simulink model "sampleModel7126_pp_1_1"  (R2018a)
settings: Solver=VariableStepAuto  StartTime=0.0  StopTime=10.0  RelTol=1e-3
undefined symbols (not defined in the file): DiscIntNeverNeededParam
libraries: simulink x367
(part 12 of 12)

== system sampleModel7126_pp_1_1/cfblk284/cfblk10/emi_600 ==
  Action Port : ActionPort  ActionType=else
  emi_601 : Assertion

== system sampleModel7126_pp_1_1/cfblk284/cfblk11/cfblk10 ==
  emi_481 : Inport
  emi_482 : Inport  Port=2
  Action Port : ActionPort  ActionType=then
  cfblk10 : simulink/Continuous/PID Controller (2DOF)  Controller=PID  TimeDomain=Discrete-time  SampleTime=-1  IntegratorMethod=Forward Euler  FilterMethod=Forward Euler  Form=Parallel  UseFilter=on  ControllerParametersSource=internal  P=1  I=1  D=0  N=100  b=1  c=1  InitialConditionSource=internal  InitialConditionForIntegrator=0  InitialConditionForFilter=0  ExternalReset=none  LimitOutput=off  UpperSaturationLimit=inf  LowerSaturationLimit=-inf  LinearizeAsGain=off  AntiWindupMode=none  Kb=1  TrackingMode=off  Kt=1  PParamMin=[]  PParamMax=[]  IParamMin=[]  IParamMax=[]  DParamMin=[]  DParamMax=[]  NParamMin=[]  NParamMax=[]  bParamMin=[]  bParamMax=[]  cParamMin=[]  cParamMax=[]  KbParamMin=[]  KbParamMax=[]  KtParamMin=[]  KtParamMax=[]  POutMin=[]  POutMax=[]  IOutMin=[]  IOutMax=[]  DOutMin=[]  DOutMax=[]  NOutMin=[]  NOutMax=[]  bOutMin=[]  bOutMax=[]  cOutMin=[]  cOutMax=[]  KbOutMin=[]  KbOutMax=[]  KtOutMin=[]  KtOutMax=[]  IntegratorOutMin=[]  IntegratorOutMax=[]  FilterOutMin=[]  FilterOutMax=[]  SumOutMin=[]  SumOutMax=[]  Sum1OutMin=[]  Sum1OutMax=[]  Sum2OutMin=[]  Sum2OutMax=[]  Sum3OutMin=[]  Sum3OutMax=[]  SumI1OutMin=[]  SumI1OutMax=[]  SumI2OutMin=[]  SumI2OutMax=[]  SumI3OutMin=[]  SumI3OutMax=[]  SumDOutMin=[]  SumDOutMax=[]  SaturationOutMin=[]  SaturationOutMax=[]  IntegratorContinuousStateAttributes=''  IntegratorStateMustResolveToSignalObject=off  IntegratorRTWStateStorageClass=Auto  FilterContinuousStateAttributes=''  FilterStateMustResolveToSignalObject=off  FilterRTWStateStorageClass=Auto  DifferentiatorICPrevScaledInput=0  DifferentiatorOutMin=[]  DifferentiatorOutMax=[]  FilterDiffOutCoefMin=[]  FilterDiffOutCoefMax=[]  SumDenOutMin=[]  SumDenOutMax=[]  SumNumOutMin=[]  SumNumOutMax=[]  ReciprocalOutMin=[]  ReciprocalOutMax=[]  DivideOutMin=[]  DivideOutMax=[]  TunerSelectOption=Transfer Function Based (PID Tuner App)
  emi_483 : Outport
  wires:
  emi_481/1 -> cfblk10/1
  emi_482/1 -> cfblk10/2
  cfblk10/1 -> emi_483/1

== system sampleModel7126_pp_1_1/cfblk284/cfblk11/cfblk11 ==
  emi_1583 : Inport
  Action Port : ActionPort  ActionType=then
  cfblk11 : simulink/Discrete/Transfer Fcn Real Zero  ZeroZ=0.75  ICPrevInput=0.0  DoSatur=off
      settings: SourceProductName=Simulink  SourceProductBaseCode=SL
  emi_1584 : Outport
  wires:
  emi_1583/1 -> cfblk11/1
  cfblk11/1 -> emi_1584/1

== system sampleModel7126_pp_1_1/cfblk284/cfblk11/cfblk4 ==
  emi_1611 : Inport
  Action Port : ActionPort  ActionType=then
  cfblk4 : simulink/Discrete/Transfer Fcn Real Zero  ZeroZ=0.75  ICPrevInput=0.0  DoSatur=off
      settings: SourceProductName=Simulink  SourceProductBaseCode=SL
  emi_1612 : Outport
  wires:
  emi_1611/1 -> cfblk4/1
  cfblk4/1 -> emi_1612/1

== system sampleModel7126_pp_1_1/cfblk284/cfblk11/cfblk8 ==
  emi_1461 : Inport
  emi_1462 : Inport  Port=2
  Action Port : ActionPort  ActionType=then
  cfblk8 : simulink/Continuous/PID Controller (2DOF)  Controller=PID  TimeDomain=Discrete-time  SampleTime=-1  IntegratorMethod=Forward Euler  FilterMethod=Forward Euler  Form=Parallel  UseFilter=on  ControllerParametersSource=internal  P=1  I=1  D=0  N=100  b=1  c=1  InitialConditionSource=internal  InitialConditionForIntegrator=0  InitialConditionForFilter=0  ExternalReset=none  LimitOutput=off  UpperSaturationLimit=inf  LowerSaturationLimit=-inf  LinearizeAsGain=off  AntiWindupMode=none  Kb=1  TrackingMode=off  Kt=1  PParamMin=[]  PParamMax=[]  IParamMin=[]  IParamMax=[]  DParamMin=[]  DParamMax=[]  NParamMin=[]  NParamMax=[]  bParamMin=[]  bParamMax=[]  cParamMin=[]  cParamMax=[]  KbParamMin=[]  KbParamMax=[]  KtParamMin=[]  KtParamMax=[]  POutMin=[]  POutMax=[]  IOutMin=[]  IOutMax=[]  DOutMin=[]  DOutMax=[]  NOutMin=[]  NOutMax=[]  bOutMin=[]  bOutMax=[]  cOutMin=[]  cOutMax=[]  KbOutMin=[]  KbOutMax=[]  KtOutMin=[]  KtOutMax=[]  IntegratorOutMin=[]  IntegratorOutMax=[]  FilterOutMin=[]  FilterOutMax=[]  SumOutMin=[]  SumOutMax=[]  Sum1OutMin=[]  Sum1OutMax=[]  Sum2OutMin=[]  Sum2OutMax=[]  Sum3OutMin=[]  Sum3OutMax=[]  SumI1OutMin=[]  SumI1OutMax=[]  SumI2OutMin=[]  SumI2OutMax=[]  SumI3OutMin=[]  SumI3OutMax=[]  SumDOutMin=[]  SumDOutMax=[]  SaturationOutMin=[]  SaturationOutMax=[]  IntegratorContinuousStateAttributes=''  IntegratorStateMustResolveToSignalObject=off  IntegratorRTWStateStorageClass=Auto  FilterContinuousStateAttributes=''  FilterStateMustResolveToSignalObject=off  FilterRTWStateStorageClass=Auto  DifferentiatorICPrevScaledInput=0  DifferentiatorOutMin=[]  DifferentiatorOutMax=[]  FilterDiffOutCoefMin=[]  FilterDiffOutCoefMax=[]  SumDenOutMin=[]  SumDenOutMax=[]  SumNumOutMin=[]  SumNumOutMax=[]  ReciprocalOutMin=[]  ReciprocalOutMax=[]  DivideOutMin=[]  DivideOutMax=[]  TunerSelectOption=Transfer Function Based (PID Tuner App)
  emi_1463 : Outport
  wires:
  emi_1461/1 -> cfblk8/1
  emi_1462/1 -> cfblk8/2
  cfblk8/1 -> emi_1463/1

== system sampleModel7126_pp_1_1/cfblk284/cfblk11/emi_1464 ==
  Action Port : ActionPort  ActionType=else
  emi_1465 : Assertion

== system sampleModel7126_pp_1_1/cfblk284/cfblk11/emi_1585 ==
  Action Port : ActionPort  ActionType=else
  emi_1586 : Assertion

== system sampleModel7126_pp_1_1/cfblk284/cfblk11/emi_1613 ==
  Action Port : ActionPort  ActionType=else
  emi_1614 : Assertion

== system sampleModel7126_pp_1_1/cfblk284/cfblk11/emi_484 ==
  Action Port : ActionPort  ActionType=else
  emi_485 : Assertion

== system sampleModel7126_pp_1_1/cfblk289/cfblk10/cfblk4 ==
  emi_981 : Inport
  Action Port : ActionPort  ActionType=then
  cfblk4 : DiscreteIntegrator  SampleTime=-1  OutDataTypeStr=double  ICPrevOutput=DiscIntNeverNeededParam  ICPrevScaledInput=DiscIntNeverNeededParam
  emi_982 : Outport
  wires:
  emi_981/1 -> cfblk4/1
  cfblk4/1 -> emi_982/1

== system sampleModel7126_pp_1_1/cfblk289/cfblk10/cfblk5 ==
  emi_974 : Inport
  Action Port : ActionPort  ActionType=then
  cfblk5 : simulink/Discrete/Transfer Fcn Real Zero  ZeroZ=0.75  ICPrevInput=0.0  DoSatur=off
      settings: SourceProductName=Simulink  SourceProductBaseCode=SL
  emi_975 : Outport
  wires:
  emi_974/1 -> cfblk5/1
  cfblk5/1 -> emi_975/1

== system sampleModel7126_pp_1_1/cfblk289/cfblk10/cfblk7 ==
  emi_1405 : Inport
  Action Port : ActionPort  ActionType=then
  cfblk7 : Delay
  emi_1406 : Outport
  wires:
  emi_1405/1 -> cfblk7/1
  cfblk7/1 -> emi_1406/1

== system sampleModel7126_pp_1_1/cfblk289/cfblk10/cfblk9 ==
  emi_584 : Inport
  Action Port : ActionPort  ActionType=then
  cfblk9 : DiscreteFilter
  emi_585 : Outport
  wires:
  emi_584/1 -> cfblk9/1
  cfblk9/1 -> emi_585/1

== system sampleModel7126_pp_1_1/cfblk289/cfblk10/emi_1407 ==
  Action Port : ActionPort  ActionType=else
  emi_1408 : Assertion

== system sampleModel7126_pp_1_1/cfblk289/cfblk10/emi_586 ==
  Action Port : ActionPort  ActionType=else
  emi_587 : Assertion

== system sampleModel7126_pp_1_1/cfblk289/cfblk10/emi_976 ==
  Action Port : ActionPort  ActionType=else
  emi_977 : Assertion

== system sampleModel7126_pp_1_1/cfblk289/cfblk10/emi_983 ==
  Action Port : ActionPort  ActionType=else
  emi_984 : Assertion

== system sampleModel7126_pp_1_1/cfblk289/cfblk9/cfblk10 ==
  emi_818 : Inport
  Action Port : ActionPort  ActionType=then
  cfblk10 : DiscreteFir
  emi_819 : Outport
  wires:
  emi_818/1 -> cfblk10/1
  cfblk10/1 -> emi_819/1

== system sampleModel7126_pp_1_1/cfblk289/cfblk9/cfblk12 ==
  emi_1667 : Inport
  Action Port : ActionPort  ActionType=then
  cfblk12 : DiscreteTransferFcn
  emi_1668 : Outport
  wires:
  emi_1667/1 -> cfblk12/1
  cfblk12/1 -> emi_1668/1

== system sampleModel7126_pp_1_1/cfblk289/cfblk9/cfblk15 ==
  emi_1246 : Inport
  emi_1247 : Inport  Port=2
  Action Port : ActionPort  ActionType=then
  cfblk15 : simulink/Continuous/PID Controller (2DOF)  Controller=PID  TimeDomain=Discrete-time  SampleTime=-1  IntegratorMethod=Forward Euler  FilterMethod=Forward Euler  Form=Parallel  UseFilter=on  ControllerParametersSource=internal  P=1  I=1  D=0  N=100  b=1  c=1  InitialConditionSource=internal  InitialConditionForIntegrator=0  InitialConditionForFilter=0  ExternalReset=none  LimitOutput=off  UpperSaturationLimit=inf  LowerSaturationLimit=-inf  LinearizeAsGain=off  AntiWindupMode=none  Kb=1  TrackingMode=off  Kt=1  PParamMin=[]  PParamMax=[]  IParamMin=[]  IParamMax=[]  DParamMin=[]  DParamMax=[]  NParamMin=[]  NParamMax=[]  bParamMin=[]  bParamMax=[]  cParamMin=[]  cParamMax=[]  KbParamMin=[]  KbParamMax=[]  KtParamMin=[]  KtParamMax=[]  POutMin=[]  POutMax=[]  IOutMin=[]  IOutMax=[]  DOutMin=[]  DOutMax=[]  NOutMin=[]  NOutMax=[]  bOutMin=[]  bOutMax=[]  cOutMin=[]  cOutMax=[]  KbOutMin=[]  KbOutMax=[]  KtOutMin=[]  KtOutMax=[]  IntegratorOutMin=[]  IntegratorOutMax=[]  FilterOutMin=[]  FilterOutMax=[]  SumOutMin=[]  SumOutMax=[]  Sum1OutMin=[]  Sum1OutMax=[]  Sum2OutMin=[]  Sum2OutMax=[]  Sum3OutMin=[]  Sum3OutMax=[]  SumI1OutMin=[]  SumI1OutMax=[]  SumI2OutMin=[]  SumI2OutMax=[]  SumI3OutMin=[]  SumI3OutMax=[]  SumDOutMin=[]  SumDOutMax=[]  SaturationOutMin=[]  SaturationOutMax=[]  IntegratorContinuousStateAttributes=''  IntegratorStateMustResolveToSignalObject=off  IntegratorRTWStateStorageClass=Auto  FilterContinuousStateAttributes=''  FilterStateMustResolveToSignalObject=off  FilterRTWStateStorageClass=Auto  DifferentiatorICPrevScaledInput=0  DifferentiatorOutMin=[]  DifferentiatorOutMax=[]  FilterDiffOutCoefMin=[]  FilterDiffOutCoefMax=[]  SumDenOutMin=[]  SumDenOutMax=[]  SumNumOutMin=[]  SumNumOutMax=[]  ReciprocalOutMin=[]  ReciprocalOutMax=[]  DivideOutMin=[]  DivideOutMax=[]  TunerSelectOption=Transfer Function Based (PID Tuner App)
  emi_1248 : Outport
  wires:
  emi_1246/1 -> cfblk15/1
  emi_1247/1 -> cfblk15/2
  cfblk15/1 -> emi_1248/1

== system sampleModel7126_pp_1_1/cfblk289/cfblk9/cfblk8 ==
  emi_1433 : Inport
  Action Port : ActionPort  ActionType=then
  cfblk8 : Delay
  emi_1434 : Outport
  wires:
  emi_1433/1 -> cfblk8/1
  cfblk8/1 -> emi_1434/1

== system sampleModel7126_pp_1_1/cfblk289/cfblk9/cfblk9 ==
  emi_1254 : Inport
  Action Port : ActionPort  ActionType=then
  cfblk9 : DiscreteFir
  emi_1255 : Outport
  wires:
  emi_1254/1 -> cfblk9/1
  cfblk9/1 -> emi_1255/1

== system sampleModel7126_pp_1_1/cfblk289/cfblk9/emi_1249 ==
  Action Port : ActionPort  ActionType=else
  emi_1250 : Assertion

== system sampleModel7126_pp_1_1/cfblk289/cfblk9/emi_1256 ==
  Action Port : ActionPort  ActionType=else
  emi_1257 : Assertion

== system sampleModel7126_pp_1_1/cfblk289/cfblk9/emi_1435 ==
  Action Port : ActionPort  ActionType=else
  emi_1436 : Assertion

== system sampleModel7126_pp_1_1/cfblk289/cfblk9/emi_1669 ==
  Action Port : ActionPort  ActionType=else
  emi_1670 : Assertion

== system sampleModel7126_pp_1_1/cfblk289/cfblk9/emi_820 ==
  Action Port : ActionPort  ActionType=else
  emi_821 : Assertion

== system sampleModel7126_pp_1_1/cfblk292/cfblk14/cfblk3 ==
  emi_1426 : Inport
  Action Port : ActionPort  ActionType=then
  cfblk3 : DiscreteFir
  emi_1427 : Outport
  wires:
  emi_1426/1 -> cfblk3/1
  cfblk3/1 -> emi_1427/1

== system sampleModel7126_pp_1_1/cfblk292/cfblk14/cfblk4 ==
  emi_351 : Inport
  Action Port : ActionPort  ActionType=then
  cfblk4 : simulink/Discrete/Transfer Fcn Real Zero  ZeroZ=0.75  ICPrevInput=0.0  DoSatur=off
      settings: SourceProductName=Simulink  SourceProductBaseCode=SL
  emi_352 : Outport
  wires:
  emi_351/1 -> cfblk4/1
  cfblk4/1 -> emi_352/1

== system sampleModel7126_pp_1_1/cfblk292/cfblk14/emi_1428 ==
  Action Port : ActionPort  ActionType=else
  emi_1429 : Assertion

== system sampleModel7126_pp_1_1/cfblk292/cfblk14/emi_353 ==
  Action Port : ActionPort  ActionType=else
  emi_354 : Assertion

== system sampleModel7126_pp_1_1/cfblk292/cfblk15/cfblk13 ==
  emi_1412 : Inport
  Action Port : ActionPort  ActionType=then
  cfblk13 : Delay
  emi_1413 : Outport
  wires:
  emi_1412/1 -> cfblk13/1
  cfblk13/1 -> emi_1413/1

== system sampleModel7126_pp_1_1/cfblk292/cfblk15/cfblk3 ==
  emi_453 : Inport
  Action Port : ActionPort  ActionType=then
  cfblk3 : simulink/Continuous/PID Controller  Controller=PID  TimeDomain=Discrete-time  SampleTime=-1  IntegratorMethod=Forward Euler  FilterMethod=Forward Euler  Form=Parallel  UseFilter=on  ControllerParametersSource=internal  P=1  I=1  D=0  N=100  InitialConditionSource=internal  InitialConditionForIntegrator=0  InitialConditionForFilter=0  ExternalReset=none  LimitOutput=off  UpperSaturationLimit=inf  LowerSaturationLimit=-inf  LinearizeAsGain=off  AntiWindupMode=none  Kb=1  TrackingMode=off  Kt=1  PParamMin=[]  PParamMax=[]  IParamMin=[]  IParamMax=[]  DParamMin=[]  DParamMax=[]  NParamMin=[]  NParamMax=[]  KbParamMin=[]  KbParamMax=[]  KtParamMin=[]  KtParamMax=[]  POutMin=[]  POutMax=[]  IOutMin=[]  IOutMax=[]  DOutMin=[]  DOutMax=[]  NOutMin=[]  NOutMax=[]  KbOutMin=[]  KbOutMax=[]  KtOutMin=[]  KtOutMax=[]  IntegratorOutMin=[]  IntegratorOutMax=[]  FilterOutMin=[]  FilterOutMax=[]  SumOutMin=[]  SumOutMax=[]  SumI1OutMin=[]  SumI1OutMax=[]  SumI2OutMin=[]  SumI2OutMax=[]  SumI3OutMin=[]  SumI3OutMax=[]  SumDOutMin=[]  SumDOutMax=[]  SaturationOutMin=[]  SaturationOutMax=[]  IntegratorContinuousStateAttributes=''  IntegratorStateMustResolveToSignalObject=off  IntegratorRTWStateStorageClass=Auto  FilterContinuousStateAttributes=''  FilterStateMustResolveToSignalObject=off  FilterRTWStateStorageClass=Auto  DifferentiatorICPrevScaledInput=0  DifferentiatorOutMin=[]  DifferentiatorOutMax=[]  FilterDiffOutCoefMin=[]  FilterDiffOutCoefMax=[]  SumDenOutMin=[]  SumDenOutMax=[]  SumNumOutMin=[]  SumNumOutMax=[]  ReciprocalOutMin=[]  ReciprocalOutMax=[]  DivideOutMin=[]  DivideOutMax=[]  TunerSelectOption=Transfer Function Based (PID Tuner App)
  emi_454 : Outport
  wires:
  emi_453/1 -> cfblk3/1
  cfblk3/1 -> emi_454/1

== system sampleModel7126_pp_1_1/cfblk292/cfblk15/cfblk5 ==
  emi_1762 : Inport
  Action Port : ActionPort  ActionType=then
  cfblk5 : DiscreteStateSpace  SampleTime=-1
  emi_1763 : Outport
  wires:
  emi_1762/1 -> cfblk5/1
  cfblk5/1 -> emi_1763/1

== system sampleModel7126_pp_1_1/cfblk292/cfblk15/cfblk6 ==
  emi_1732 : Inport
  emi_1733 : Inport  Port=2
  Action Port : ActionPort  ActionType=then
  cfblk6 : simulink/Continuous/PID Controller (2DOF)  Controller=PID  TimeDomain=Discrete-time  SampleTime=-1  IntegratorMethod=Forward Euler  FilterMethod=Forward Euler  Form=Parallel  UseFilter=on  ControllerParametersSource=internal  P=1  I=1  D=0  N=100  b=1  c=1  InitialConditionSource=internal  InitialConditionForIntegrator=0  InitialConditionForFilter=0  ExternalReset=none  LimitOutput=off  UpperSaturationLimit=inf  LowerSaturationLimit=-inf  LinearizeAsGain=off  AntiWindupMode=none  Kb=1  TrackingMode=off  Kt=1  PParamMin=[]  PParamMax=[]  IParamMin=[]  IParamMax=[]  DParamMin=[]  DParamMax=[]  NParamMin=[]  NParamMax=[]  bParamMin=[]  bParamMax=[]  cParamMin=[]  cParamMax=[]  KbParamMin=[]  KbParamMax=[]  KtParamMin=[]  KtParamMax=[]  POutMin=[]  POutMax=[]  IOutMin=[]  IOutMax=[]  DOutMin=[]  DOutMax=[]  NOutMin=[]  NOutMax=[]  bOutMin=[]  bOutMax=[]  cOutMin=[]  cOutMax=[]  KbOutMin=[]  KbOutMax=[]  KtOutMin=[]  KtOutMax=[]  IntegratorOutMin=[]  IntegratorOutMax=[]  FilterOutMin=[]  FilterOutMax=[]  SumOutMin=[]  SumOutMax=[]  Sum1OutMin=[]  Sum1OutMax=[]  Sum2OutMin=[]  Sum2OutMax=[]  Sum3OutMin=[]  Sum3OutMax=[]  SumI1OutMin=[]  SumI1OutMax=[]  SumI2OutMin=[]  SumI2OutMax=[]  SumI3OutMin=[]  SumI3OutMax=[]  SumDOutMin=[]  SumDOutMax=[]  SaturationOutMin=[]  SaturationOutMax=[]  IntegratorContinuousStateAttributes=''  IntegratorStateMustResolveToSignalObject=off  IntegratorRTWStateStorageClass=Auto  FilterContinuousStateAttributes=''  FilterStateMustResolveToSignalObject=off  FilterRTWStateStorageClass=Auto  DifferentiatorICPrevScaledInput=0  DifferentiatorOutMin=[]  DifferentiatorOutMax=[]  FilterDiffOutCoefMin=[]  FilterDiffOutCoefMax=[]  SumDenOutMin=[]  SumDenOutMax=[]  SumNumOutMin=[]  SumNumOutMax=[]  ReciprocalOutMin=[]  ReciprocalOutMax=[]  DivideOutMin=[]  DivideOutMax=[]  TunerSelectOption=Transfer Function Based (PID Tuner App)
  emi_1734 : Outport
  wires:
  emi_1732/1 -> cfblk6/1
  emi_1733/1 -> cfblk6/2
  cfblk6/1 -> emi_1734/1

== system sampleModel7126_pp_1_1/cfblk292/cfblk15/emi_1414 ==
  Action Port : ActionPort  ActionType=else
  emi_1415 : Assertion

== system sampleModel7126_pp_1_1/cfblk292/cfblk15/emi_1735 ==
  Action Port : ActionPort  ActionType=else
  emi_1736 : Assertion

== system sampleModel7126_pp_1_1/cfblk292/cfblk15/emi_1764 ==
  Action Port : ActionPort  ActionType=else
  emi_1765 : Assertion

== system sampleModel7126_pp_1_1/cfblk292/cfblk15/emi_455 ==
  Action Port : ActionPort  ActionType=else
  emi_456 : Assertion

== system sampleModel7126_pp_1_1/cfblk295/cfblk13/cfblk5 ==
  emi_988 : Inport
  Action Port : ActionPort  ActionType=then
  cfblk5 : simulink/Discrete/Transfer Fcn Real Zero  ZeroZ=0.75  ICPrevInput=0.0  DoSatur=off
      settings: SourceProductName=Simulink  SourceProductBaseCode=SL
  emi_989 : Outport
  wires:
  emi_988/1 -> cfblk5/1
  cfblk5/1 -> emi_989/1

== system sampleModel7126_pp_1_1/cfblk295/cfblk13/emi_990 ==
  Action Port : ActionPort  ActionType=else
  emi_991 : Assertion

== system sampleModel7126_pp_1_1/cfblk295/cfblk14/cfblk11 ==
  emi_422 : Inport
  Action Port : ActionPort  ActionType=then
  cfblk11 : simulink/Continuous/PID Controller  Controller=PID  TimeDomain=Discrete-time  SampleTime=-1  IntegratorMethod=Forward Euler  FilterMethod=Forward Euler  Form=Parallel  UseFilter=on  ControllerParametersSource=internal  P=1  I=1  D=0  N=100  InitialConditionSource=internal  InitialConditionForIntegrator=0  InitialConditionForFilter=0  ExternalReset=none  LimitOutput=off  UpperSaturationLimit=inf  LowerSaturationLimit=-inf  LinearizeAsGain=off  AntiWindupMode=none  Kb=1  TrackingMode=off  Kt=1  PParamMin=[]  PParamMax=[]  IParamMin=[]  IParamMax=[]  DParamMin=[]  DParamMax=[]  NParamMin=[]  NParamMax=[]  KbParamMin=[]  KbParamMax=[]  KtParamMin=[]  KtParamMax=[]  POutMin=[]  POutMax=[]  IOutMin=[]  IOutMax=[]  DOutMin=[]  DOutMax=[]  NOutMin=[]  NOutMax=[]  KbOutMin=[]  KbOutMax=[]  KtOutMin=[]  KtOutMax=[]  IntegratorOutMin=[]  IntegratorOutMax=[]  FilterOutMin=[]  FilterOutMax=[]  SumOutMin=[]  SumOutMax=[]  SumI1OutMin=[]  SumI1OutMax=[]  SumI2OutMin=[]  SumI2OutMax=[]  SumI3OutMin=[]  SumI3OutMax=[]  SumDOutMin=[]  SumDOutMax=[]  SaturationOutMin=[]  SaturationOutMax=[]  IntegratorContinuousStateAttributes=''  IntegratorStateMustResolveToSignalObject=off  IntegratorRTWStateStorageClass=Auto  FilterContinuousStateAttributes=''  FilterStateMustResolveToSignalObject=off  FilterRTWStateStorageClass=Auto  DifferentiatorICPrevScaledInput=0  DifferentiatorOutMin=[]  DifferentiatorOutMax=[]  FilterDiffOutCoefMin=[]  FilterDiffOutCoefMax=[]  SumDenOutMin=[]  SumDenOutMax=[]  SumNumOutMin=[]  SumNumOutMax=[]  ReciprocalOutMin=[]  ReciprocalOutMax=[]  DivideOutMin=[]  DivideOutMax=[]  TunerSelectOption=Transfer Function Based (PID Tuner App)
  emi_423 : Outport
  wires:
  emi_422/1 -> cfblk11/1
  cfblk11/1 -> emi_423/1

== system sampleModel7126_pp_1_1/cfblk295/cfblk14/cfblk12 ==
  emi_1210 : Inport
  Action Port : ActionPort  ActionType=then
  cfblk12 : simulink/Discrete/Tapped Delay  vinit=0.0  samptime=-1  NumDelays=1  DelayOrder=Oldest  includeCurrent=off
  emi_1211 : Outport
  wires:
  emi_1210/1 -> cfblk12/1
  cfblk12/1 -> emi_1211/1

== system sampleModel7126_pp_1_1/cfblk295/cfblk14/cfblk6 ==
  emi_1362 : Inport
  Action Port : ActionPort  ActionType=then
  cfblk6 : DiscreteZeroPole  Poles=[0 0.5]  Gain=1  SampleTime=-1
  emi_1363 : Outport
  wires:
  emi_1362/1 -> cfblk6/1
  cfblk6/1 -> emi_1363/1

== system sampleModel7126_pp_1_1/cfblk295/cfblk14/cfblk7 ==
  emi_1799 : Inport
  Action Port : ActionPort  ActionType=then
  cfblk7 : simulink/Discrete/Tapped Delay  vinit=0.0  samptime=-1  NumDelays=1  DelayOrder=Oldest  includeCurrent=off
  emi_1800 : Outport
  wires:
  emi_1799/1 -> cfblk7/1
  cfblk7/1 -> emi_1800/1

== system sampleModel7126_pp_1_1/cfblk295/cfblk14/emi_1212 ==
  Action Port : ActionPort  ActionType=else
  emi_1213 : Assertion

== system sampleModel7126_pp_1_1/cfblk295/cfblk14/emi_1364 ==
  Action Port : ActionPort  ActionType=else
  emi_1365 : Assertion

== system sampleModel7126_pp_1_1/cfblk295/cfblk14/emi_1801 ==
  Action Port : ActionPort  ActionType=else
  emi_1802 : Assertion

== system sampleModel7126_pp_1_1/cfblk295/cfblk14/emi_424 ==
  Action Port : ActionPort  ActionType=else
  emi_425 : Assertion

== system sampleModel7126_pp_1_1/cfblk298/cfblk15/cfblk4 ==
  emi_1682 : Inport
  Action Port : ActionPort  ActionType=then
  cfblk4 : DiscreteFilter
  emi_1683 : Outport
  wires:
  emi_1682/1 -> cfblk4/1
  cfblk4/1 -> emi_1683/1

== system sampleModel7126_pp_1_1/cfblk298/cfblk15/cfblk5 ==
  emi_633 : Inport
  Action Port : ActionPort  ActionType=then
  cfblk5 : DiscreteFir
  emi_634 : Outport
  wires:
  emi_633/1 -> cfblk5/1
  cfblk5/1 -> emi_634/1

== system sampleModel7126_pp_1_1/cfblk298/cfblk15/cfblk7 ==
  emi_2066 : Inport
  Action Port : ActionPort  ActionType=then
  cfblk7 : Delay
  emi_2067 : Outport
  wires:
  emi_2066/1 -> cfblk7/1
  cfblk7/1 -> emi_2067/1

== system sampleModel7126_pp_1_1/cfblk298/cfblk15/cfblk9 ==
  emi_2022 : Inport
  Action Port : ActionPort  ActionType=then
  cfblk9 : simulink/Discrete/Tapped Delay  vinit=0.0  samptime=-1  NumDelays=1  DelayOrder=Oldest  includeCurrent=off
  emi_2023 : Outport
  wires:
  emi_2022/1 -> cfblk9/1
  cfblk9/1 -> emi_2023/1

== system sampleModel7126_pp_1_1/cfblk298/cfblk15/emi_1684 ==
  Action Port : ActionPort  ActionType=else
  emi_1685 : Assertion

== system sampleModel7126_pp_1_1/cfblk298/cfblk15/emi_2024 ==
  Action Port : ActionPort  ActionType=else
  emi_2025 : Assertion

== system sampleModel7126_pp_1_1/cfblk298/cfblk15/emi_2068 ==
  Action Port : ActionPort  ActionType=else
  emi_2069 : Assertion

== system sampleModel7126_pp_1_1/cfblk298/cfblk15/emi_635 ==
  Action Port : ActionPort  ActionType=else
  emi_636 : Assertion

== system sampleModel7126_pp_1_1/cfblk298/cfblk16/cfblk10 ==
  emi_1813 : Inport
  Action Port : ActionPort  ActionType=then
  cfblk10 : DiscreteTransferFcn
  emi_1814 : Outport
  wires:
  emi_1813/1 -> cfblk10/1
  cfblk10/1 -> emi_1814/1

== system sampleModel7126_pp_1_1/cfblk298/cfblk16/cfblk6 ==
  emi_903 : Inport
  Action Port : ActionPort  ActionType=then
  cfblk6 : simulink/Discrete/Transfer Fcn Real Zero  ZeroZ=0.75  ICPrevInput=0.0  DoSatur=off
      settings: SourceProductName=Simulink  SourceProductBaseCode=SL
  emi_904 : Outport
  wires:
  emi_903/1 -> cfblk6/1
  cfblk6/1 -> emi_904/1

== system sampleModel7126_pp_1_1/cfblk298/cfblk16/cfblk8 ==
  emi_1447 : Inport
  Action Port : ActionPort  ActionType=then
  cfblk8 : simulink/Discrete/Tapped Delay  vinit=0.0  samptime=-1  NumDelays=1  DelayOrder=Oldest  includeCurrent=off
  emi_1448 : Outport
  wires:
  emi_1447/1 -> cfblk8/1
  cfblk8/1 -> emi_1448/1

== system sampleModel7126_pp_1_1/cfblk298/cfblk16/emi_1449 ==
  Action Port : ActionPort  ActionType=else
  emi_1450 : Assertion

== system sampleModel7126_pp_1_1/cfblk298/cfblk16/emi_1815 ==
  Action Port : ActionPort  ActionType=else
  emi_1816 : Assertion

== system sampleModel7126_pp_1_1/cfblk298/cfblk16/emi_905 ==
  Action Port : ActionPort  ActionType=else
  emi_906 : Assertion
